simulink model "ADCS_r2017b"  (R2018a)
settings: Solver=FixedStepAuto  StartTime=0.0  StopTime=end_time  FixedStep=delta_t  RelTol=1e-3
undefined symbols (not defined in the file or in its folder): delta_t, SC, SS
libraries: sharedutil x5, vrlib x2
(part 2 of 3)

== system ADCS_r2017b/Satellite Simulator/Kinematics/Position Kinematics/Adams Bashforth Integration2 ==
  x_initial : Inport
  x_dot : Inport  Port=2
  dt : Inport  Port=3
  Delay : Delay  DelayLength=1  InitialConditionSource=Input port  InitialCondition=0
      settings: InputPortMap=u0,p4
  Delay1 : Delay  DelayLength=1  InitialConditionSource=Input port  InitialCondition=0
      settings: InputPortMap=u0,p4
  Delay2 : Delay  DelayLength=1  InitialConditionSource=Input port  InitialCondition=0
      settings: InputPortMap=u0,p4
  Gain : Gain  Gain=23/12
  Gain1 : Gain  Gain=-16/12
  Gain2 : Gain  Gain=5/12
  Product : Product
  Sum : Sum  Inputs=|++
  Sum1 : Sum  Inputs=+++
  x : Outport
  wires:
  x_initial/1 -> Delay/2
  Delay/1 -> Sum/1
  Sum/1 -> Delay/1, x/1
  Delay1/1 -> Delay2/1, Gain1/1
  x_dot/1 -> Delay2/2, Delay1/2, Delay1/1, Gain/1
  Gain1/1 -> Sum1/2
  Gain/1 -> Sum1/1
  Gain2/1 -> Sum1/3
  Sum1/1 -> Product/1
  dt/1 -> Product/2
  Product/1 -> Sum/2
  Delay2/1 -> Gain2/1

== system ADCS_r2017b/Satellite Simulator/Kinematics/Rotation Kinematics/Adams Bashforth Integration ==
  x_initial : Inport
  x_dot : Inport  Port=2
  dt : Inport  Port=3
  Delay : Delay  DelayLength=1  InitialConditionSource=Input port  InitialCondition=0
      settings: InputPortMap=u0,p4
  Delay1 : Delay  DelayLength=1  InitialConditionSource=Input port  InitialCondition=0
      settings: InputPortMap=u0,p4
  Delay2 : Delay  DelayLength=1  InitialConditionSource=Input port  InitialCondition=0
      settings: InputPortMap=u0,p4
  Gain : Gain  Gain=23/12
  Gain1 : Gain  Gain=-16/12
  Gain2 : Gain  Gain=5/12
  Product : Product
  Quaternion Normalize : sharedutil/Quaternion Normalize
      settings: SourceProductName=Aerospace Blockset  SourceProductBaseCode=AE
  Sum : Sum  Inputs=|++
  Sum1 : Sum  Inputs=+++
  x : Outport
  wires:
  x_initial/1 -> Delay/2
  Delay/1 -> Sum/1
  Sum/1 -> Quaternion Normalize/1
  Delay1/1 -> Delay2/1, Gain1/1
  x_dot/1 -> Delay2/2, Delay1/2, Delay1/1, Gain/1
  Gain1/1 -> Sum1/2
  Gain/1 -> Sum1/1
  Gain2/1 -> Sum1/3
  Sum1/1 -> Product/1
  dt/1 -> Product/2
  Product/1 -> Sum/2
  Delay2/1 -> Gain2/1
  Quaternion Normalize/1 -> Delay/1, x/1

== system ADCS_r2017b/Satellite Simulator/Kinematics/Rotation Kinematics/Adams Bashforth Integration1 ==
  x_initial : Inport
  x_dot : Inport  Port=2
  dt : Inport  Port=3
  Delay : Delay  DelayLength=1  InitialConditionSource=Input port  InitialCondition=0
      settings: InputPortMap=u0,p4
  Delay1 : Delay  DelayLength=1  InitialConditionSource=Input port  InitialCondition=0
      settings: InputPortMap=u0,p4
  Delay2 : Delay  DelayLength=1  InitialConditionSource=Input port  InitialCondition=0
      settings: InputPortMap=u0,p4
  Gain : Gain  Gain=23/12
  Gain1 : Gain  Gain=-16/12
  Gain2 : Gain  Gain=5/12
  Product : Product
  Sum : Sum  Inputs=|++
  Sum1 : Sum  Inputs=+++
  x : Outport
  wires:
  x_initial/1 -> Delay/2
  Delay/1 -> Sum/1
  Sum/1 -> Delay/1, x/1
  Delay1/1 -> Delay2/1, Gain1/1
  x_dot/1 -> Delay2/2, Delay1/2, Delay1/1, Gain/1
  Gain1/1 -> Sum1/2
  Gain/1 -> Sum1/1
  Gain2/1 -> Sum1/3
  Sum1/1 -> Product/1
  dt/1 -> Product/2
  Product/1 -> Sum/2
  Delay2/1 -> Gain2/1

== system ADCS_r2017b/Flight Software/Subsystems/RCS Controller/3 Axis Controller/Controller ==
  q_est : Inport
  w_est : Inport  Port=2
  q_target : Inport  Port=3
  w_target : Inport  Port=4
  gains : Inport  Port=5
  Constant : Constant  Value=[0;0;0;0;0;0;0;0;0;0;0;0]
  Terminator{,1..4} (5 alike) : Terminator
  RCS Cmd : Outport
  wires:
  q_est/1 -> Terminator/1
  w_est/1 -> Terminator1/1
  q_target/1 -> Terminator2/1
  w_target/1 -> Terminator3/1
  Constant/1 -> RCS Cmd/1
  gains/1 -> Terminator4/1

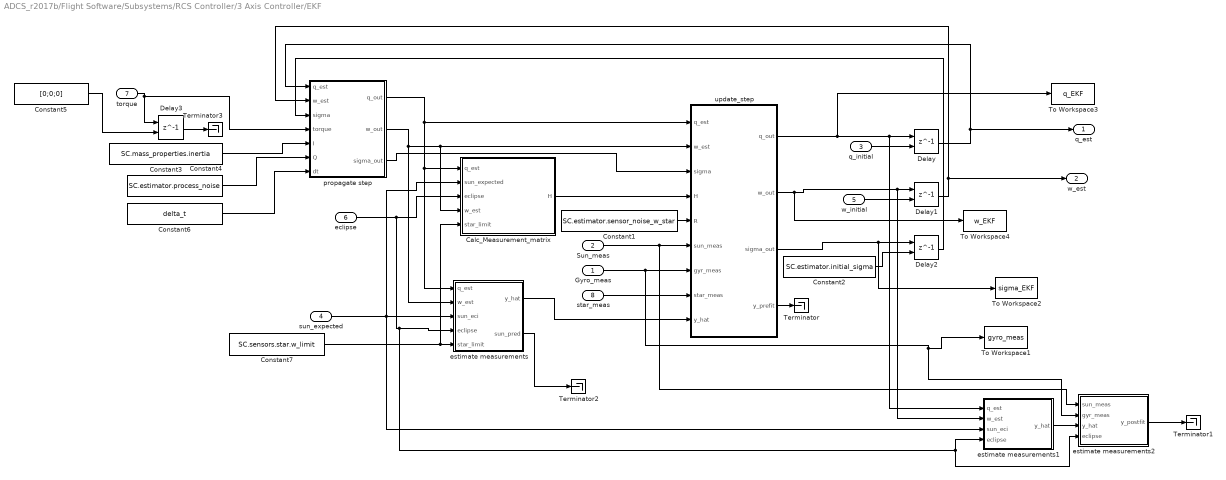
== system ADCS_r2017b/Flight Software/Subsystems/RCS Controller/3 Axis Controller/EKF ==
  Gyro_meas : Inport
  Sun_meas : Inport  Port=2
  q_initial : Inport  Port=3
  sun_expected : Inport  Port=4
  w_initial : Inport  Port=5
  eclipse : Inport  Port=6
  torque : Inport  Port=7
  star_meas : Inport  Port=8
  Calc_Measurement_matrix : MATLAB Function  TreatAsAtomicUnit=on
  Constant1 : Constant  Value=SC.estimator.sensor_noise_w_star
  Constant2 : Constant  Value=SC.estimator.initial_sigma
  Constant3 : Constant  Value=SC.mass_properties.inertia
  Constant4 : Constant  Value=SC.estimator.process_noise
  Constant5 : Constant  Value=[0;0;0]
  Constant6 : Constant  Value=delta_t
  Constant7 : Constant  Value=SC.sensors.star.w_limit
  Delay{,1..3} (4 alike) : Delay  DelayLength=1  InitialConditionSource=Input port  InitialCondition=0
      settings: InputPortMap=u0,p4
  Terminator{,1..3} (4 alike) : Terminator
  To Workspace1 : ToWorkspace  VariableName=gyro_meas  SampleTime=-1
  To Workspace2 : ToWorkspace  VariableName=sigma_EKF  SampleTime=-1
  To Workspace3 : ToWorkspace  VariableName=q_EKF  SampleTime=-1
  To Workspace4 : ToWorkspace  VariableName=w_EKF  SampleTime=-1
  estimate measurements : MATLAB Function  TreatAsAtomicUnit=on
  estimate measurements1 : MATLAB Function  TreatAsAtomicUnit=on
  estimate measurements2 : MATLAB Function  TreatAsAtomicUnit=on
  propagate step : MATLAB Function  TreatAsAtomicUnit=on
  update_step : MATLAB Function  TreatAsAtomicUnit=on
  q_est : Outport
  w_est : Outport  Port=2
  wires:
  Constant3/1 -> propagate step/5(I)
  sun_expected/1 -> estimate measurements/3(sun_eci), Calc_Measurement_matrix/2(sun_expected), estimate measurements1/3(sun_eci)
  Delay2/1 -> propagate step/3(sigma)
  Constant6/1 -> propagate step/7(dt)
  estimate measurements/1(y_hat) -> update_step/9(y_hat)
  q_initial/1 -> Delay/2
  estimate measurements2/1(y_postfit) -> Terminator1/1
  eclipse/1 -> estimate measurements/4(eclipse), estimate measurements1/4(eclipse), estimate measurements2/4(eclipse), Calc_Measurement_matrix/3(eclipse)
  update_step/2(w_out) -> To Workspace4/1, estimate measurements1/2(w_est), Delay1/1
  Delay1/1 -> w_est/1, propagate step/2(w_est)
  Constant4/1 -> propagate step/6(Q)
  update_step/1(q_out) -> To Workspace3/1, estimate measurements1/1(q_est), Delay/1
  w_initial/1 -> Delay1/2
  propagate step/2(w_out) -> Calc_Measurement_matrix/4(w_est), update_step/2(w_est), estimate measurements/2(w_est)
  propagate step/1(q_out) -> update_step/1(q_est), estimate measurements/1(q_est), Calc_Measurement_matrix/1(q_est)
  estimate measurements/2(sun_pred) -> Terminator2/1
  Delay/1 -> q_est/1, propagate step/1(q_est)
  Constant1/1 -> update_step/5(R)
  Calc_Measurement_matrix/1(H) -> update_step/4(H)
  Constant2/1 -> Delay2/2
  propagate step/3(sigma_out) -> update_step/3(sigma)
  Sun_meas/1 -> estimate measurements2/1(sun_meas), update_step/6(sun_meas)
  update_step/3(sigma_out) -> To Workspace2/1, Delay2/1
  Gyro_meas/1 -> To Workspace1/1, estimate measurements2/2(gyr_meas), update_step/7(gyr_meas)
  estimate measurements1/1(y_hat) -> estimate measurements2/3(y_hat)
  torque/1 -> propagate step/4(torque), Delay3/1
  Constant5/1 -> Delay3/2
  Constant7/1 -> Calc_Measurement_matrix/5(star_limit), estimate measurements/5(star_limit)
  star_meas/1 -> update_step/8(star_meas)
  update_step/4(y_prefit) -> Terminator/1
  Delay3/1 -> Terminator3/1

== system ADCS_r2017b/Flight Software/Subsystems/RCS Controller/3 Axis Controller/State Estimator ==
  gyro : Inport
  sun : Inport  Port=2
  star : Inport  Port=3
  Sun_eci_expected : Inport  Port=4
  Deterministic : Subsystem
  Q Method : Subsystem
  Subsystem : Subsystem
  To Workspace : ToWorkspace  VariableName=q_est_det  SampleTime=-1
  To Workspace1 : ToWorkspace  VariableName=w_est_det  SampleTime=-1
  To Workspace2 : ToWorkspace  VariableName=q_est_q  SampleTime=-1
  To Workspace3 : ToWorkspace  VariableName=w_est_q  SampleTime=-1
  To Workspace4 : ToWorkspace  VariableName=q_est_int  SampleTime=-1
  To Workspace5 : ToWorkspace  VariableName=w_est_int  SampleTime=-1
  q_est : Outport
  w_est : Outport  Port=2
  wires:
  gyro/1 -> Subsystem/1(w_body), Q Method/2(gyro), Deterministic/1(gyro)
  star/1 -> Q Method/3(star), Deterministic/2(star)
  sun/1 -> Q Method/1(sun_dir)
  Deterministic/1(q_est) -> To Workspace/1
  Deterministic/2(w_est) -> To Workspace1/1
  Q Method/1(q_est) -> To Workspace2/1, q_est/1
  Q Method/2(w_est) -> To Workspace3/1, w_est/1
  Subsystem/1(q_est) -> To Workspace4/1
  Subsystem/2(w_est) -> To Workspace5/1
  Sun_eci_expected/1 -> Q Method/4(sun_exp)

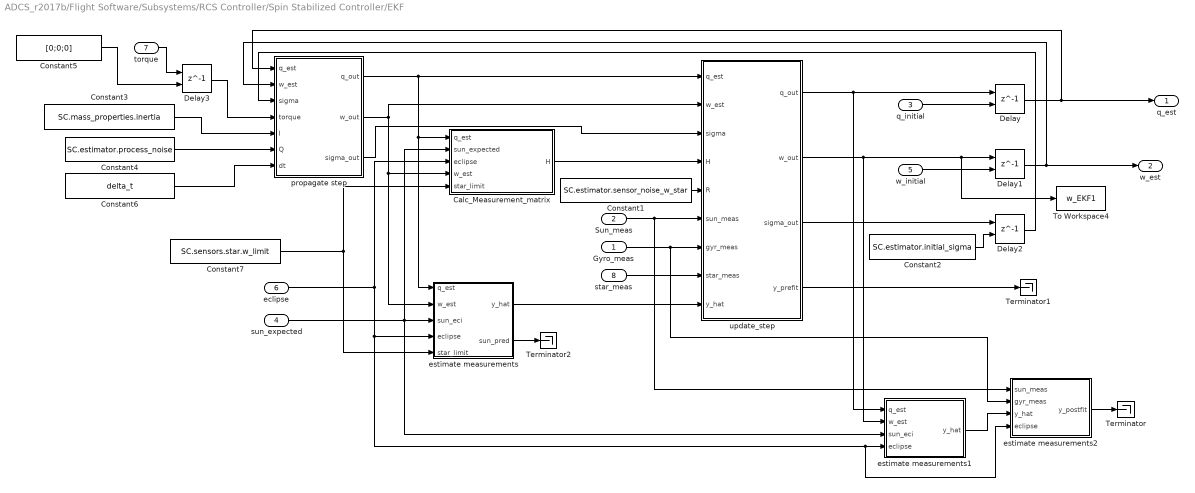
== system ADCS_r2017b/Flight Software/Subsystems/RCS Controller/Spin Stabilized Controller/EKF ==
  Gyro_meas : Inport
  Sun_meas : Inport  Port=2
  q_initial : Inport  Port=3
  sun_expected : Inport  Port=4
  w_initial : Inport  Port=5
  eclipse : Inport  Port=6
  torque : Inport  Port=7
  star_meas : Inport  Port=8
  Calc_Measurement_matrix : MATLAB Function  TreatAsAtomicUnit=on
  Constant1 : Constant  Value=SC.estimator.sensor_noise_w_star
  Constant2 : Constant  Value=SC.estimator.initial_sigma
  Constant3 : Constant  Value=SC.mass_properties.inertia
  Constant4 : Constant  Value=SC.estimator.process_noise
  Constant5 : Constant  Value=[0;0;0]
  Constant6 : Constant  Value=delta_t
  Constant7 : Constant  Value=SC.sensors.star.w_limit
  Delay{,1..3} (4 alike) : Delay  DelayLength=1  InitialConditionSource=Input port  InitialCondition=0
      settings: InputPortMap=u0,p4
  Terminator : Terminator
  Terminator1 : Terminator
  Terminator2 : Terminator
  To Workspace4 : ToWorkspace  VariableName=w_EKF1  SampleTime=-1
  estimate measurements : MATLAB Function  TreatAsAtomicUnit=on
  estimate measurements1 : MATLAB Function  TreatAsAtomicUnit=on
  estimate measurements2 : MATLAB Function  TreatAsAtomicUnit=on
  propagate step : MATLAB Function  TreatAsAtomicUnit=on
  update_step : MATLAB Function  TreatAsAtomicUnit=on
  q_est : Outport
  w_est : Outport  Port=2
  wires:
  Constant3/1 -> propagate step/5(I)
  sun_expected/1 -> Calc_Measurement_matrix/2(sun_expected), estimate measurements/3(sun_eci), estimate measurements1/3(sun_eci)
  Delay2/1 -> propagate step/3(sigma)
  Constant6/1 -> propagate step/7(dt)
  estimate measurements/1(y_hat) -> update_step/9(y_hat)
  q_initial/1 -> Delay/2
  estimate measurements2/1(y_postfit) -> Terminator/1
  eclipse/1 -> Calc_Measurement_matrix/3(eclipse), estimate measurements2/4(eclipse), estimate measurements1/4(eclipse), estimate measurements/4(eclipse)
  update_step/2(w_out) -> estimate measurements1/2(w_est), To Workspace4/1, Delay1/1
  Delay1/1 -> propagate step/2(w_est), w_est/1
  Constant4/1 -> propagate step/6(Q)
  update_step/4(y_prefit) -> Terminator1/1
  update_step/1(q_out) -> estimate measurements1/1(q_est), Delay/1
  w_initial/1 -> Delay1/2
  propagate step/2(w_out) -> update_step/2(w_est), Calc_Measurement_matrix/4(w_est), estimate measurements/2(w_est)
  propagate step/1(q_out) -> update_step/1(q_est), estimate measurements/1(q_est), Calc_Measurement_matrix/1(q_est)
  Delay/1 -> propagate step/1(q_est), q_est/1
  Constant1/1 -> update_step/5(R)
  Calc_Measurement_matrix/1(H) -> update_step/4(H)
  Constant2/1 -> Delay2/2
  propagate step/3(sigma_out) -> update_step/3(sigma)
  Sun_meas/1 -> update_step/6(sun_meas), estimate measurements2/1(sun_meas)
  update_step/3(sigma_out) -> Delay2/1
  Gyro_meas/1 -> update_step/7(gyr_meas), estimate measurements2/2(gyr_meas)
  estimate measurements1/1(y_hat) -> estimate measurements2/3(y_hat)
  Delay3/1 -> propagate step/4(torque)
  torque/1 -> Delay3/1
  Constant5/1 -> Delay3/2
  estimate measurements/2(sun_pred) -> Terminator2/1
  star_meas/1 -> update_step/8(star_meas)
  Constant7/1 -> estimate measurements/5(star_limit), Calc_Measurement_matrix/5(star_limit)

== system ADCS_r2017b/Flight Software/Subsystems/RCS Controller/3 Axis Controller/State Estimator/Deterministic ==
  gyro : Inport
  star : Inport  Port=2
  q_est : Outport
  w_est : Outport  Port=2
  wires:
  star/1 -> q_est/1
  gyro/1 -> w_est/1

== system ADCS_r2017b/Flight Software/Subsystems/RCS Controller/3 Axis Controller/State Estimator/Q Method ==
  sun_dir : Inport
  gyro : Inport  Port=2
  star : Inport  Port=3
  sun_exp : Inport  Port=4
  Constant : Constant  Value=SC.sensors.weights
  q_method : MATLAB Function  TreatAsAtomicUnit=on
  q_est : Outport  PortDimensions=4
  w_est : Outport  Port=2
  wires:
  sun_dir/1 -> q_method/2(sun_meas)
  q_method/1(q) -> q_est/1
  gyro/1 -> w_est/1
  star/1 -> q_method/3(q_body)
  sun_exp/1 -> q_method/1(sun_expected)
  Constant/1 -> q_method/4(weights)

== system ADCS_r2017b/Flight Software/Subsystems/RCS Controller/3 Axis Controller/State Estimator/Subsystem ==
  w_body : Inport
  Adams Bashforth Integration : Subsystem  TreatAsAtomicUnit=on
  Constant : Constant  Value=SC.initial_state.q
  Constant2 : Constant  Value=delta_t
  Delay : Delay  DelayLength=1  InitialConditionSource=Input port  InitialCondition=0
      settings: InputPortMap=u0,p4
  calc_q_dot : MATLAB Function  TreatAsAtomicUnit=on
  q_est : Outport
  w_est : Outport  Port=2
  wires:
  calc_q_dot/1(q_dot) -> Adams Bashforth Integration/2(x_dot)
  w_body/1 -> w_est/1, calc_q_dot/2(w)
  Constant/1 -> Delay/2, Adams Bashforth Integration/1(x_initial)
  Delay/1 -> calc_q_dot/1(q)
  Constant2/1 -> Adams Bashforth Integration/3(dt)
  Adams Bashforth Integration/1(x) -> Delay/1, q_est/1

== system ADCS_r2017b/Flight Software/Subsystems/RCS Controller/3 Axis Controller/State Estimator/Subsystem/Adams Bashforth Integration ==
  x_initial : Inport
  x_dot : Inport  Port=2
  dt : Inport  Port=3
  Delay : Delay  DelayLength=1  InitialConditionSource=Input port  InitialCondition=0
      settings: InputPortMap=u0,p4
  Delay1 : Delay  DelayLength=1  InitialConditionSource=Input port  InitialCondition=0
      settings: InputPortMap=u0,p4
  Delay2 : Delay  DelayLength=1  InitialConditionSource=Input port  InitialCondition=0
      settings: InputPortMap=u0,p4
  Gain : Gain  Gain=23/12
  Gain1 : Gain  Gain=-16/12
  Gain2 : Gain  Gain=5/12
  Product : Product
  Quaternion Normalize : sharedutil/Quaternion Normalize
      settings: SourceProductName=Aerospace Blockset  SourceProductBaseCode=AE
  Sum : Sum  Inputs=|++
  Sum1 : Sum  Inputs=+++
  x : Outport
  wires:
  x_initial/1 -> Delay/2
  Delay/1 -> Sum/1
  Sum/1 -> Quaternion Normalize/1
  Delay1/1 -> Delay2/1, Gain1/1
  x_dot/1 -> Delay2/2, Delay1/2, Delay1/1, Gain/1
  Gain1/1 -> Sum1/2
  Gain/1 -> Sum1/1
  Gain2/1 -> Sum1/3
  Sum1/1 -> Product/1
  dt/1 -> Product/2
  Product/1 -> Sum/2
  Delay2/1 -> Gain2/1
  Quaternion Normalize/1 -> Delay/1, x/1

== matlab function ADCS_r2017b/Flight Software/Subsystems/Sensor Processing/Process Gyro ==
  data: raw input; gyro output; gain input; offset input; rot input
function gyro = process_gyro(raw, gain, offset, rot)

temp = rot * raw;
gyro = gain .* (temp - offset);

== matlab function ADCS_r2017b/Flight Software/Subsystems/Mode Selection/MATLAB Function ==
  data: Kp output; gyro input; Kd output; eclipse input; JD input; mode output; ax3_gains input; ax3_TC input; spin_gains input; spin_TC input; spin_up_gains input; spin_up_TC input
function [Kp, Kd, mode]  = Mode_Logic(gyro, eclipse, JD, ax3_gains, ax3_TC, spin_gains, spin_TC, spin_up_gains, spin_up_TC)
%JD_i = 2458610.000; %initial JD
JD_i = 2458611.2081011; %actual initial JD
minutes_elapsed = (JD-JD_i)*(24*60);

if(minutes_elapsed < 10)
    mode = 0; %de-tumble controller
elseif(minutes_elapsed < 20)
    mode = 1; %three axis control
elseif(minutes_elapsed < 30)
    mode = 3; %spin controller
else
    mode = 4; %uncontrolled
end

if mode == 0
    Kp = 0*ax3_gains(1:3);
    Kd = ax3_gains(4:6);
elseif mode == 1
    Kp = ax3_gains(1:3);
    Kd = ax3_gains(4:6);
elseif mode == 2
    Kp = spin_up_gains(1:3);
    Kd = spin_up_gains(4:6);
elseif mode == 3
    Kp = spin_gains(1:3);
    Kd = spin_gains(4:6);
else
    Kp = [0;0;0];
    Kd = [0;0;0];
end
    
end

== matlab function ADCS_r2017b/Flight Software/Subsystems/Sensor Processing/Process Gyro1 ==
  data: raw input; sun_dir output; gain input; offset input; eclipse output; threshold input
function [sun_dir, eclipse] = process_sun(raw, gain, offset, threshold)
n = length(raw); %number of sun sensors
sun = zeros(n,1);
for i=1:length(raw)
    sun(i) = gain(i) * (raw(i) - offset(i));
end

%discuss advantages of different ways of turning sun measurements to direction
sun_x = sun(1)-sun(2);
sun_y = sun(3)-sun(4);
sun_z = sun(5)-sun(6);

sun_dir = [sun_x; sun_y; sun_z];
sun_dir = sun_dir/norm(sun_dir);

eclipse = 0;
if (sum(abs(sun)) < threshold)
    eclipse = 1;
    sun_dir = [0;0;0];
end

== matlab function ADCS_r2017b/Satellite Simulator/Kinematics/Backup Rotation Kinematics/Euler Equations ==
  data: w input; w_dot output; tor input; I input
function w_dot = fcn(w, tor, I)

w_dot = -I\(Skew(w)*I*w-tor);

% w_dot = zeros(size(w));
% wx = w(1); wy = w(2); wz = w(3);
% Ix = I(1,1); Iy = I(2,2); Iz = I(3,3);
% w_dot(1) = (tor(1) - (Iz-Iy)*wx*wz)/Ix;  %update this to work in body axis
% w_dot(2) = (tor(2) - (Ix-Iz)*wz*wx)/Iy;
% w_dot(3) = (tor(3) - (Iy-Ix)*wx*wy)/Iz;
end


function S = Skew(v)
S = [0 -v(3) v(2)
    v(3) 0 -v(1)
    -v(2) v(1) 0];
end

== matlab function ADCS_r2017b/Satellite Simulator/Kinematics/Backup Rotation Kinematics/calc_e_dot ==
  data: e input; e_dot output; w input
function e_dot   = calc_e_dot( e, w )
%INPUT: euler angles, angular velocity
%OUTPUT: rate of change of euler angles
%propagate actual dynamics
    tan_the = tan(e(2));
    if(abs(tan_the) > 300) %make sure tan(theta) is well defined
        tan_the = 300*sign(tan_the);
        disp('tan x')
    end
    cos_the = cos(e(2));
    if(abs(cos_the) < 10^-4) %make sure cos(theta) is well defined
        cos_the = 10^-4*sign(cos_the);
        disp('cos x')
    end
    A = [1, tan_the*sin(e(1)), tan_the*cos(e(1));
         0, cos(e(1)),              -1*sin(e(1));
         0, sin(e(1))/cos_the,  cos(e(1))/cos_the];
    e_dot = A*w;
end

== matlab function ADCS_r2017b/Satellite Simulator/External Forces and Torques/External Forces/MATLAB Function ==
  data: srp input; srp_tot output
function srp_tot = fcn(srp)
%srp_tot = zeros(3,1);
%srp is 3x6
srp_tot = sum(srp, 2);
%srp_tot = [0;0;0];

== matlab function ADCS_r2017b/Satellite Simulator/Kinematics/Calc Coordinate Transforms/Calc_R_eci2body ==
  data: q input; R_eci2body output
function R_eci2body = fcn(q)
eta=q(4);
e1=q(1);
e2=q(2);
e3=q(3);

R_eci2body = [e1^2-e2^2-e3^2+eta^2, 2*(e1*e2+eta*e3),        2*(e1*e3-eta*e2);
              2*(e1*e2-eta*e3),     -1*e1^2+e2^2-e3^2+eta^2, 2*(e2*e3+eta*e1);
              2*(e1*e3+eta*e2),     2*(e2*e3-eta*e1),        -1*e1^2-e2^2+e3^2+eta^2];
          
end

== matlab function ADCS_r2017b/Satellite Simulator/External Forces and Torques/External Torques/MATLAB Function ==
  data: r_mci input; y output; r_moon input
function y = fcn(r_mci, r_moon)

y = (norm(r_mci) < 0.9*r_moon);

== matlab function ADCS_r2017b/Satellite Simulator/Kinematics/Calc Coordinate Transforms/Calc_R_eci2ecef ==
  data: JD_i input; R_eci2ecef output
function R_eci2ecef = fcn(JD_i)
%Based on Seidlemann's "Explanatory Supplment to the Astronomical Almanac" page 50
%Given the JD, will return the rotation matrix to convert R_eci to R_ecef
JD = floor(JD_i);
seconds_per_day = 24*60*60;
SSN = seconds_per_day*(JD_i-JD);
seconds_per_half_day = seconds_per_day/2;
days_per_Julian_century = 36525;
JD_epoch = 2451545.00; %JD of noon on Jan 1, 2000

c1 = JD-JD_epoch+(SSN/seconds_per_day);
c2 = c1/days_per_Julian_century;

p1 = 24110.54841;
p2 = 8640184.812866;
p3 = 0.093104;
p4 = -6.2*10^-6;

c3 = (p1)+(p2*c2)+(p3*c2*c2)+(p4*c2*c2*c2)+(SSN)-(seconds_per_half_day);

c4 = c3*pi/seconds_per_half_day;

c5 = mod(c4, 2*pi);

a1 = cos(c5);
a2 = sin(c5);
a3 = -1*a2;
a4 = 0;
a5 = 1;
A = [a1;a3;a4;a2;a1;a4;a4;a4;a5];

R_eci2ecef = reshape(A, 3,3);
end

== matlab function ADCS_r2017b/Satellite Simulator/Kinematics/Calc Coordinate Transforms/ecef2geod ==
  data: h output; r_ecef input; phi output; lambda output
function [h,phi,lambda] = ecef2geod(r_ecef)
%note - r_ecef should be in meters
a = 6378137;        %earth radius, meters
e = 0.081819190842; %earth eccentricity

% Reference: function ecef2geodetic in Matlab
x = r_ecef(1);
y = r_ecef(2);
z = r_ecef(3);

% Ellipsoid constants
e2 = e ^ 2;   % Square of first eccentricity
ep2 = e2 / (1 - e2);     % Square of second eccentricity
f = 1 - sqrt(1 - e2);    % Flattening
b = a * (1 - f);         % Semiminor axis
% Longitude
lambda = atan2(y,x); %[rad]
% Distance from Z-axis
rho = hypot(x,y);
% Bowring's formula for initial parametric (beta) and geodetic (phi) latitudes
beta = atan2(z, (1 - f) * rho);
phi = atan2(z   + b * ep2 * sin(beta).^3,...
            rho - a * e2  * cos(beta).^3); %[rad]
% Fixed-point iteration with Bowring's formula
% (typically converges within two or three iterations)
betaNew = atan2((1 - f)*sin(phi), cos(phi));
count = 0;
while any(beta ~= betaNew) && count < 5
    beta = betaNew;
    phi = atan2(z   + b * ep2 * sin(beta).^3,...
                rho - a * e2  * cos(beta).^3);
    betaNew = atan2((1 - f)*sin(phi), cos(phi));
    count = count + 1;
end
% Calculate ellipsoidal height from the final value for latitude
sinphi = sin(phi);
N = a ./ sqrt(1 - e2 * sinphi.^2);
h = rho .* cos(phi) + (z + e2 * N .* sinphi) .* sinphi - N;

phi=phi*180/pi; %[deg]
lambda=lambda*180/pi; %[deg]
end

== matlab function ADCS_r2017b/Satellite Simulator/Kinematics/Rotation Kinematics/calc_q_dot ==
  data: q input; q_dot output; w input
function q_dot   = fcn(q, w)

wx = w(1); wy = w(2); wz = w(3);
OMEGA = [   0,    wz, -1*wy, wx;
        -1*wz,     0,    wx, wy;
           wy, -1*wx,     0, wz;
        -1*wx, -1*wy, -1*wz,  0];
q_dot = 0.5*OMEGA*q;

== matlab function ADCS_r2017b/Satellite Simulator/Environment/Subsystem/MATLAB Function ==
  data: decYear input; B_ned output; yearLastEpoch input; lastgh input; ghslope input; latitude input; longitude input; altitude input
function B_ned  = igrf_mag_field(decYear, yearLastEpoch, lastgh, ghslope, latitude, longitude, altitude)
% IGRF Earth's magnetic field from IGRF model.
% 
% Usage: B = IGRF(COEFS, LATITUDE, LONGITUDE, ALTITUDE)
% 
% Calculates the components of the Earth's magnetic field using the
% International Geomagnetic Reference Field (IGRF) model. The inputs for
% the position can be scalars.
% 
% When all the coordinate inputs are scalars, the function can be run more
% efficiently by providing the proper IGRF coefficient vector for a given
% time rather than the time itself. This mode is useful when making
% multiple calls to the function while keeping the time the same (meaning
% the coefficients will be the same for each run) as loading the
% coefficients can be the most time-consuming part of the function. The
% coefficient vector can be easily loaded using the function LOADIGRFCOEFS.
% This mode is assumed when all the coordinate inputs are scalars and the
% first input is a vector. In this case, the coefficient vector should be
% formatted as (LOADIGRFCOEFS provides this):
% 
%   [g(n=1,m=0) g(n=1,m=1) h(n=1,m=1) g(n=2,m=0) g(n=2,m=1) h(n=2,m=1) ...]
% 
% Regardless of the size of the inputs, the outputs will be column vectors.
% If only one output is requested, B = [BX(:), BY(:), BZ(:)] is output.
% Note that the other parameters the IGRF gives can be computed from BX,
% BY, and BZ as:
% 
%   Horizonal intensity: hypot(BX, BY) (i.e., sqrt(BX.^2 + BY.^2) )
%   Total intensity: hypot(BX, hypot(BY, BZ))
%   Declination: atan2(BY, BX)
%   Inclination: atan(BZ./hypot(BX, BY))
% 
% This function relies on having the file igrfcoefs.mat in the MATLAB
% path to function properly when a time is input. If this file cannot be
% found, this function will try to create it by calling GETIGRFCOEFS.
% 
% The IGRF is a spherical harmonic expansion of the Earth's internal
% magnetic field. Currently, the IGRF model is valid between the years 1900
% and 2015. See the health warning for the IGRF model here:
% http://www.ngdc.noaa.gov/IAGA/vmod/igrfhw.html
% 
% Reference:
% International Association of Geomagnetism and Aeronomy, Working Group 
% V-MOD (2010), International Geomagnetic Reference Field: the eleventh
% generation, _Geophys. J. Int._, _183_(3), 1216-1230, 
% doi:10.1111/j.1365-246X.2010.04804.x.
% 
% Inputs:
%   -COEFS: Instead of inputting a time, you can simply specify the proper
%   coefficients for the time you want by inputting in the first argument
%   the proper coefficient vector from igrfcoefs.mat.
%   -LATITUDE: Geocentric or geodetic latitude in degrees.
%   -LONGITUDE: Geocentric or geodetic longitude in degrees.
%   -ALTITUDE: For geodetic coordiates, the height in km above the Earth's
%   surface. For geocentric coordiates, the radius in km from the center of
%   the Earth.

% 
% Outputs:
%   -BX: Northward component of the magnetic field in nanoteslas (nT).
%   -BY: Eastward component of the magnetic field in nT.
%   -BZ: Downward component of the magnetic field in nT.
%   -B: [BX(:), BY(:), BZ(:)].
% 
% See also: LOADIGRFCOEFS, GETIGRFCOEFS, IGRFLINE, DATENUM, IGRF11MAGM.


%%%%%%%%%%%%%%%%%%%%%%%%%%%%%%%%%%%%%%%%%%%%%%%%%%%%%%%%%%%%%%%%%%%%%%%%%%%
%%%%%%%%%%%%%%%%%%%        IGRF scalar function.        %%%%%%%%%%%%%%%%%%%
%%%%%%%%%%%%%%%%%%%%%%%%%%%%%%%%%%%%%%%%%%%%%%%%%%%%%%%%%%%%%%%%%%%%%%%%%%%
%function [Bx, By, Bz] = igrfs(time, latitude, longitude, altitude, coord)

% Fundamental constant.
Rearth_km = 6371.2;
altitude=altitude/1000;
%%% SPHERICAL COORDINATE CONVERSION %%%
% Convert the latitude, longitude, and altitude coordinates input into
% spherical coordinates r (radius), theta (inclination angle from +z axis),
% and phi (azimuth angle from +x axis).
% We want cos(theta) and sin(theta) rather than theta itself.
costheta = cos((90 - latitude)*pi/180);
sintheta = sin((90 - latitude)*pi/180);

% Convert from geodetic coordinates to geocentric coordinates if necessary.
% This method was adapted from igrf11syn, which was a conversion of the
% IGRF subroutine written in FORTRAN.

    a = 6378.137; f = 1/298.257223563; b = a*(1 - f);
    rho = hypot(a*sintheta, b*costheta);
    r = sqrt( altitude.^2 + 2*altitude.*rho + ...
        (a^4*sintheta.^2 + b^4*costheta.^2) ./ rho.^2 );
    cd = (altitude + rho) ./ r;
    sd = (a^2 - b^2) ./ rho .* costheta.*sintheta./r;
    oldcos = costheta;
    costheta = costheta.*cd - sintheta.*sd;
    sintheta = sintheta.*cd + oldcos.*sd;


% Convert longitude to radians.
phi = longitude*pi/180;

%%% GET PROPER IGRF COEFFICIENTS %%%

gh=lastgh+ghslope*(decYear-yearLastEpoch);
nmax = sqrt(numel(gh) + 1) - 1;


% We need cos(m*phi) and sin(m*phi) multiple times, so precalculate into a
% vector here:
cosphi = cos((1:nmax)*phi);
sinphi = sin((1:nmax)*phi);

Pmax = (nmax+1)*(nmax+2)/2;

%%% BEGIN MAGNETIC FIELD CALCULATION %%%
% Initialize variables used in for loop below.
Br = 0; Bt = 0; Bp = 0;
 P = zeros(1, Pmax);  P(1) = 1;  P(3) = sintheta;
dP = zeros(1, Pmax); dP(1) = 0; dP(3) = costheta;

% For this initial condition, the first if will result in n = 1, m = 0.
m = 1; n = 0; coefindex = 1;

a_r = (Rearth_km/r)^2;

% Increment through all the n's and m's. gh will be a vector with g
% followed by h for incrementing through n and m except when h would be
% redundant (i.e., when m = 0).
for Pindex = 2:Pmax
    
    % Increment to the next n when m becomes larger than n.
    if n < m
        m = 0;
        n = n + 1;
        a_r = a_r*(Rearth_km/r); % We need (Rearth_km./r)^(n+2)
    end
    
    % Calculate P and dP. They are given recursively according to:
    % 
    % P(0, 0) = 1, P(1, 1) = sin(theta) <- Specified above
    % P(n, n) = sqrt(1 - 1/(2n))*sin(theta)*P(n-1, n-1)
    % P(n, m) = (2n - 1)/sqrt(n^2 - m^2)*cos(theta)*P(n-1, m) -
    %     sqrt(((n-1)^2 - m^2) / (n^2 - m^2)) * P(n-2, m)
    % 
    % dP(0, 0) = 0, dP(1, 1) = cos(theta) <- Specified above
    % dP(n, n) = sqrt(1 - 1/(2n))*(sin(theta)*dP(n-1, n-1) +
    %     cos(theta)*P(n-1, n-1))
    % dP(n, m) = (2n - 1)/sqrt(n^2 - m^2)*(cos(theta)*dP(n-1, m) -
    %     sin(theta)*P(n-1, m)) - sqrt(((n-1)^2 - m^2)/(n^2 - m^2))*
    %     dP(n-2, m)
    if m < n && Pindex ~= 3 % (Pindex=3 is n=1, m=1, initial cond. above)
        last1n = Pindex - n;
        last2n = Pindex - 2*n + 1;
        P(Pindex) = (2*n - 1)/sqrt(n^2 - m^2)*costheta*P(last1n) - ...
            sqrt(((n-1)^2 - m^2) / (n^2 - m^2)) * P(last2n);
        dP(Pindex) = (2*n - 1)/sqrt(n^2 - m^2)*(costheta*dP(last1n) - ...
            sintheta*P(last1n)) - sqrt(((n-1)^2 - m^2) / (n^2 - m^2)) * ...
            dP(last2n);
    elseif Pindex ~= 3
        lastn = Pindex - n - 1;
        P(Pindex) = sqrt(1 - 1/(2*m))*sintheta*P(lastn);
        dP(Pindex) = sqrt(1 - 1/(2*m))*(sintheta*dP(lastn) + ...
            costheta*P(lastn));
    end
    
    % Calculate the magnetic field components as a running sum. Find
    % explicit expressions for these in Global Earth Physics: a Handbook of
    % Physical Constants by Thomas J. Aherns (1995), pg. 49. Link:
    % http://books.google.com/books?id=aqjU_NHyre4C&lpg=PP1&dq=Global%20
    % earth%20physics%3A%20a%20handbook%20of%20physical%20constants&pg=PA49
    % #v=onepage&q&f=false
    % (except equation 6 is missing a required 1/sin(theta) and m; correct
    % equations on page 5 (equations 3a-3c) of:
    % http://hanspeterschaub.info/Papers/UnderGradStudents/
    % MagneticField.pdf)
    if m == 0 % Implies h = 0, so only coefficient in gh is g
        coef = a_r*gh(coefindex); %*cos(0*phi) = 1
        Br = Br + (n+1)*coef*P(Pindex);
        Bt = Bt - coef*dP(Pindex);
        % Bp is 0 for m = 0.
        coefindex = coefindex + 1; % Only need to skip over g this time.
    else
        coef = a_r*(gh(coefindex)*cosphi(m) + gh(coefindex+1)*sinphi(m));
        Br = Br + (n+1)*coef*P(Pindex);
        Bt = Bt - coef*dP(Pindex);
        if sintheta == 0 % Use different formula when dividing by 0.
            Bp = Bp - costheta*a_r*(-gh(coefindex)*sinphi(m) + ...
                gh(coefindex+1)*cosphi(m))*dP(Pindex);
        else
            Bp = Bp - 1/sintheta*a_r*m*(-gh(coefindex)*sinphi(m) + ...
                gh(coefindex+1)*cosphi(m))*P(Pindex);
        end
        coefindex = coefindex + 2; % Skip over g and h this time.
    end
    
    % Increment m.
    m = m + 1;
    
end

% Convert from spherical to (x,y,z) = (North,East,Down).
Bx = -Bt;
By = Bp;
Bz = -Br;

% Convert back to geodetic coordinates if necessary.
Bx_old = Bx;
Bx = Bx.*cd + Bz.*sd;
Bz = Bz.*cd - Bx_old.*sd;

B_ned = [Bx;By;Bz];

== matlab function ADCS_r2017b/Satellite Simulator/Kinematics/Calc Coordinate Transforms/MATLAB Function ==
  data: lati input; R_ecef2ned output; long input
function R_ecef2ned   = calc_ECEF_to_NED( lati, long )
%Given the latitude and longitude, returns the rotation matrix to tranform
%ECEF coordinates into NED coordinates.
%   Detailed explanation goes here
phi = lati*pi/180; %radians
lam = long*pi/180; %radians
sinp = sin(phi);
sinl = sin(lam);
cosp = cos(phi);
cosl = cos(lam);

A = zeros(3,3);
A(1,1) = -1*sinp*cosl;
A(1,2) = -1*sinp*sinl;
A(1,3) =    cosp;
A(2,1) = -1*sinl;
A(2,2) =    cosl;
A(2,3) = 0;
A(3,1) = -1*cosp*cosl;
A(3,2) = -1*cosp*sinl;
A(3,3) = -1*sinp;

R_ecef2ned = A;
end

== matlab function ADCS_r2017b/Satellite Simulator/Kinematics/Calc Coordinate Transforms/Calc_R_eci2mci ==
  data: obliq_e input; R_eci2mci output; obliq_m input
function R_eci2mci = fcn(obliq_e, obliq_m)
ang = (pi/180) * (obliq_e - obliq_m);

%check if this needs to be -1*ang
R_eci2mci = [1,0,0;
             0,cos(ang),-1*sin(ang);
             0,sin(ang),   cos(ang)];
end

== matlab function ADCS_r2017b/Satellite Simulator/External Forces and Torques/External Torques/Grav gradient earth/MATLAB Function ==
  data: rIr input; tor output; r_eci input; GM input
function tor = fcn(rIr, r_eci, GM)
r = norm(r_eci);
tor = (3*GM)/(r^3) * rIr;
end

== matlab function ADCS_r2017b/Satellite Simulator/External Forces and Torques/External Torques/Grav gradient moon/MATLAB Function ==
  data: rIr input; tor output; r_mci input; GM input
function tor = fcn(rIr, r_mci, GM)
r = norm(r_mci);
tor = (3*GM)/(r^3) * rIr;

== matlab function ADCS_r2017b/Flight Software/Subsystems/RCS Controller/3 Axis Controller/Calc_R_eci2mci ==
  data: obliq_e input; R_eci2mci output; obliq_m input
function R_eci2mci = fcn(obliq_e, obliq_m)
ang = (pi/180) * (obliq_e - obliq_m);

%check if this needs to be -1*ang
R_eci2mci = [1,0,0;
             0,cos(ang),-1*sin(ang);
             0,sin(ang),   cos(ang)];
end

== matlab function ADCS_r2017b/Satellite Simulator/Actuators/RCS Model ==
  data: command input; force_body output; torque_body output; moment_arm input; norm_dir input; max_thrust input; noise input; bias input
function [force_body, torque_body] = fcn(command, moment_arm, norm_dir, max_thrust, noise, bias)
%input: 12 commands, on range from 0-1, corresponding to which thruster to fir
 force_body = [0;0;0];
torque_body = [0;0;0];
num = length(command); %number of thrusters, should be 12.

for i=1:num
    ax = bias(i,1); ay = bias(i,2); az = bias(i,3);
    R_bias = [    1,    az, -1*ay;
              -1*az,     1,    ax;
                 ay, -1*ax,     1];
    dt = 1 + noise*randn(1,1);
     force_body =  force_body - dt*max_thrust*command(i)*R_bias*norm_dir(:,i);
    torque_body = torque_body + dt*max_thrust*command(i)*cross(R_bias*norm_dir(:,i),moment_arm(:,i));
end

== matlab function ADCS_r2017b/Flight Software/Subsystems/RCS Controller/3 Axis Controller/dcm2quat ==
  data: R_mci2eci input; q output
function q = dcm2quat(R_mci2eci)
% eta=q(4);
% e1=q(1);
% e2=q(2);
% e3=q(3);
% 
% R_eci2body = [e1^2-e2^2-e3^2+eta^2, 2*(e1*e2+eta*e3),        2*(e1*e3-eta*e2);
%               2*(e1*e2-eta*e3),     -1*e1^2+e2^2-e3^2+eta^2, 2*(e2*e3+eta*e1);
%               2*(e1*e3+eta*e2),     2*(e2*e3-eta*e1),        -1*e1^2-e2^2+e3^2+eta^2];
   
A = R_mci2eci;
%q_temp = zeros(4,1);
%q_temp = dcm2quat(R_mci2eci);
%q = [q_temp(2:4), q_temp(1)]';
q4 = 0.5*sqrt(1+A(1,1) + A(2,2) + A(3,3));
q1 = (A(2,3) - A(3,2))/(4*q4);
q2 = (A(3,1) - A(1,3))/(4*q4);
q3 = (A(1,2) - A(2,1))/(4*q4);
q = [q1;q2;q3;q4];
end

== matlab function ADCS_r2017b/Flight Software/Subsystems/RCS Controller/Environment/Sun position in ECI ==
  data: JD_tt input; sun_eci output; moon_eci input; sol_emb_eph_coeff input; sol_sun_eph_coeff input; sol_sun_jd_lookup input
function sun_eci   = calc_sun_pos(JD_tt, moon_eci, sol_emb_eph_coeff, sol_sun_eph_coeff, sol_sun_jd_lookup)
%calculate the position of the sun in the eci frame based on the lookup
%coefficients and table provided.
persistent coeff2;
persistent fract_v2;

if(JD_tt > sol_sun_jd_lookup(end))
    disp('Error, JD is past final sun table value.')
end

%index and fraction of JD
k = -1;
f = -1;
for(i=1:length(sol_sun_jd_lookup-1))
    if(JD_tt >= sol_sun_jd_lookup(i) && JD_tt <= sol_sun_jd_lookup(i+1))
        k = i;
        f = (JD_tt-sol_sun_jd_lookup(i))/(sol_sun_jd_lookup(i+1)-sol_sun_jd_lookup(i)); %f in range 0,1
        break
    end
end
f = 2*f-1; %fraction scaled in valid range -1,1
if(k<0)    %past end of table, k never reset
    k = length(sol_sun_jd_lookup)-1;
    f = 1;
end
%cheby
order = 12;
y = zeros(order+1,1);
if(isempty(coeff2))
    coeff2 = zeros(order+1, order+1);
    coeff2(1,1) = 1;
    coeff2(2,2) = 1;
    for(idx = 3:order+1)
        coeff2(idx,:) = 2*[0 coeff2(idx-1,1:end-1)]-coeff2(idx-2,:);
    end
    fract_v2 = zeros(order+1,1);
    fract_v2(1) = 1;
end

y(1) = 1;
for(ind = 2:order+1)
    fract_v2(ind) = fract_v2(ind-1)*f;
    for(sub_ind = ind:-2:1)
        y(ind) = y(ind)+fract_v2(sub_ind)*coeff2(ind,sub_ind);
    end
end
y11 = y(1:11);

coeff_x1 = sol_emb_eph_coeff(k,  1:13);
coeff_y1 = sol_emb_eph_coeff(k, 14:26);
coeff_z1 = sol_emb_eph_coeff(k, 27:39);

coeff_x2 = sol_sun_eph_coeff(k,  1:11);
coeff_y2 = sol_sun_eph_coeff(k, 12:22);
coeff_z2 = sol_sun_eph_coeff(k, 23:33);

moon_pos = 0.012150585609624*moon_eci;

sun_eci = [0;0;0];
sun_eci(1) = 1000*dot(coeff_x1, y);
sun_eci(2) = 1000*dot(coeff_y1, y);
sun_eci(3) = 1000*dot(coeff_z1, y);

sun_eci = sun_eci-moon_pos;

sun_eci(1) = 1000*dot(coeff_x2, y11)-sun_eci(1);
sun_eci(2) = 1000*dot(coeff_y2, y11)-sun_eci(2);
sun_eci(3) = 1000*dot(coeff_z2, y11)-sun_eci(3);

end

== matlab function ADCS_r2017b/Flight Software/Subsystems/RCS Controller/Environment/Moon position in ECI ==
  data: JD_tt input; moon_eci output; mop_moon_eph_coeff input; mop_moon_jd_lookup input
function moon_eci   = calc_moon_pos(JD_tt, mop_moon_eph_coeff, mop_moon_jd_lookup)
%calculate the position of the moon in the eci frame based on the lookup
%coefficients and table provided.
persistent coeff;
persistent fract_v;

if(JD_tt > mop_moon_jd_lookup(end))
    disp('Error, JD is past final moon table value.')
end

%index and fraction of JD
k = -1;
f = -1;
for(i=1:length(mop_moon_jd_lookup-1))
    if(JD_tt >= mop_moon_jd_lookup(i) && JD_tt <= mop_moon_jd_lookup(i+1))
        k = i;
        f = (JD_tt-mop_moon_jd_lookup(i))/(mop_moon_jd_lookup(i+1)-mop_moon_jd_lookup(i)); %f in range 0,1
        break
    end
end
f = 2*f-1; %fraction scaled in valid range -1,1
if(k<0)    %past end of table, k never reset
    k = length(mop_moon_jd_lookup)-1;
    f = 1;
end
%cheby
order = 12;
y = zeros(order+1,1);
if(isempty(coeff))
    coeff = zeros(order+1, order+1);
    coeff(1,1) = 1;
    coeff(2,2) = 1;
    for(idx = 3:order+1)
        coeff(idx,:) = 2*[0 coeff(idx-1,1:end-1)]-coeff(idx-2,:);
    end
    fract_v = zeros(order+1,1);
    fract_v(1) = 1;
end

y(1) = 1;
for(ind = 2:order+1)
    fract_v(ind) = fract_v(ind-1)*f;
    for(sub_ind = ind:-2:1)
        y(ind) = y(ind)+fract_v(sub_ind)*coeff(ind,sub_ind);
    end
end

coeff_x = mop_moon_eph_coeff(k,  1:13);
coeff_y = mop_moon_eph_coeff(k, 14:26);
coeff_z = mop_moon_eph_coeff(k, 27:39);

moon_eci =[0;0;0];
moon_eci(1) = 1000*dot(coeff_x, y);
moon_eci(2) = 1000*dot(coeff_y, y);
moon_eci(3) = 1000*dot(coeff_z, y);
end

== matlab function ADCS_r2017b/Flight Software/Subsystems/RCS Controller/3 Axis Controller/State Estimator/Q Method/q_method ==
  data: sun_expected input; q output; sun_meas input; q_body input; weights input
function q = fcn(sun_expected, sun_meas, q_body, weights)
%q_temp = [q_body(4), q_body(1:3)'];
%xyz_meas = quat2dcm(q_temp);
q_body = q_body / norm(q_body);
eta=q_body(4);
e1=q_body(1);
e2=q_body(2);
e3=q_body(3);

xyz_meas = [e1^2-e2^2-e3^2+eta^2, 2*(e1*e2+eta*e3),          2*(e1*e3-eta*e2);
              2*(e1*e2-eta*e3),     -1*e1^2+e2^2-e3^2+eta^2, 2*(e2*e3+eta*e1);
              2*(e1*e3+eta*e2),     2*(e2*e3-eta*e1),        -1*e1^2-e2^2+e3^2+eta^2];
x_m = xyz_meas(:,1);
y_m = xyz_meas(:,2);
z_m = xyz_meas(:,3);
x_b = [1;0;0];
y_b = [0;1;0];
z_b = [0;0;1];

s_m = sun_meas / norm(sun_meas);
s_b = sun_expected  / norm(sun_expected);
w = zeros(3,4);
w(:,1) = sqrt(weights(1)) * x_m;
w(:,2) = sqrt(weights(2)) * y_m;
w(:,3) = sqrt(weights(3)) * z_m;
w(:,4) = sqrt(weights(4)) * s_m;
u = zeros(3,4);
u(:,1) = sqrt(weights(1)) * x_b;
u(:,2) = sqrt(weights(2)) * y_b;
u(:,3) = sqrt(weights(3)) * z_b;
u(:,4) = sqrt(weights(4)) * s_b;

B = w * u';
S = B+B';
Z = [B(2,3)-B(3,2); B(3,1)-B(1,3); B(1,2)-B(2,1)];
sig = trace(B);
K = [ S-eye(3)*sig, Z;
       Z', sig];

[vec, val] = eig(K);
[~, ind] = max(max(val));
q = vec(:,ind);

== matlab function ADCS_r2017b/Flight Software/Subsystems/RCS Controller/3 Axis Controller/State Estimator/Subsystem/calc_q_dot ==
  data: q input; q_dot output; w input
function q_dot   = fcn(q, w)

wx = w(1); wy = w(2); wz = w(3);
OMEGA = [   0,    wz, -1*wy, wx;
        -1*wz,     0,    wx, wy;
           wy, -1*wx,     0, wz;
        -1*wx, -1*wy, -1*wz,  0];
q_dot = 0.5*OMEGA*q;

== matlab function ADCS_r2017b/Flight Software/Subsystems/RCS Controller/Spin Stabilized Controller/Controller ==
  data: R_mci2eci input; q_est input; tor output; w_est input; Kp input; Kd input; w_des input; mode input
function tor  = fcn(R_mci2eci, q_est, w_est, Kp, Kd, w_des, mode)
if(mode < 1.5)
    w_des = 0*w_des;
end

if(mode > 3.5)
    Kp = 0*Kp;
    Kd = 0*Kd;
end

As = quat2dcm(q_est); %aka R_eci2body
At = R_mci2eci';  %target

z_body = [0;0;1];
z_mci  = [0;0;1];
z_mci  = R_mci2eci * z_mci;
z_mci  = As * z_mci; %get z_mci in the body frame
alpha  = acos(z_mci(3) / norm(z_mci)); %dot(z_body, z_mci)
vec    = cross(z_body, z_mci/norm(z_mci));
q_tar = [vec(1)*sin(alpha/2); vec(2)*sin(alpha/2); vec(3)*sin(alpha/2); cos(alpha/2)];
At = quat2dcm(q_tar); %try this instead, AZ, 6/4/2019

%Ae = As * At';
Ae = At;

%Ae_dot = (Ae-Ae_prev)/0.1;

tor = zeros(3, 1);
% linear control for small errors
% alpha_x = Ae(2,3);
% alpha_y = Ae(3,1);
% alpha_z = Ae(1,2);
% tor(1) = -Kp*alpha_x -Kd*w_est(1);
% tor(2) = -Kp*alpha_y -Kd*w_est(2);
% tor(3) = -Kp*alpha_z -Kd*w_est(3);
%Kp = [0;0;0];
% non-linear control for larger errors

tor(1) = -Kp(1)*.5*(Ae(2,3) - Ae(3,2)) - Kd(1)*(w_est(1)-w_des(1));
tor(2) = -Kp(2)*.5*(Ae(3,1) - Ae(1,3)) - Kd(2)*(w_est(2)-w_des(2));
tor(3) = -Kp(3)*.5*(Ae(1,2) - Ae(2,1)) - Kd(3)*(w_est(3)-w_des(3));

% tor(1) = -Kp(1)*.5*(Ae(2,3) - Ae(3,2)) - Kd(1)*.5*(Ae_dot(2,3) - Ae_dot(3,2));
% tor(2) = -Kp(2)*.5*(Ae(3,1) - Ae(1,3)) - Kd(2)*.5*(Ae_dot(3,1) - Ae_dot(1,3));
% tor(3) = -Kp(3)*.5*(Ae(1,2) - Ae(2,1)) - Kd(3)*.5*(Ae_dot(1,2) - Ae_dot(2,1));
end

function R_eci2body = quat2dcm(q)
eta=q(4);
e1=q(1);
e2=q(2);
e3=q(3);

R_eci2body = [e1^2-e2^2-e3^2+eta^2, 2*(e1*e2+eta*e3),        2*(e1*e3-eta*e2);
              2*(e1*e2-eta*e3),     -1*e1^2+e2^2-e3^2+eta^2, 2*(e2*e3+eta*e1);
              2*(e1*e3+eta*e2),     2*(e2*e3-eta*e1),        -1*e1^2-e2^2+e3^2+eta^2];
          
end

function S = skew(v)
S = [0 -v(3) v(2)
    v(3) 0 -v(1)
    -v(2) v(1) 0];
end

== matlab function ADCS_r2017b/Satellite Simulator/Environment/Sun position in ECI ==
  data: JD_tt input; sun_eci output; moon_eci input; sol_emb_eph_coeff input; sol_sun_eph_coeff input; sol_sun_jd_lookup input
function sun_eci   = calc_sun_pos(JD_tt, moon_eci, sol_emb_eph_coeff, sol_sun_eph_coeff, sol_sun_jd_lookup)
%calculate the position of the sun in the eci frame based on the lookup
%coefficients and table provided.
persistent coeff2;
persistent fract_v2;

if(JD_tt > sol_sun_jd_lookup(end))
    disp('Error, JD is past final sun table value.')
end

%index and fraction of JD
k = -1;
f = -1;
for(i=1:length(sol_sun_jd_lookup-1))
    if(JD_tt >= sol_sun_jd_lookup(i) && JD_tt <= sol_sun_jd_lookup(i+1))
        k = i;
        f = (JD_tt-sol_sun_jd_lookup(i))/(sol_sun_jd_lookup(i+1)-sol_sun_jd_lookup(i)); %f in range 0,1
        break
    end
end
f = 2*f-1; %fraction scaled in valid range -1,1
if(k<0)    %past end of table, k never reset
    k = length(sol_sun_jd_lookup)-1;
    f = 1;
end
%cheby
order = 12;
y = zeros(order+1,1);
if(isempty(coeff2))
    coeff2 = zeros(order+1, order+1);
    coeff2(1,1) = 1;
    coeff2(2,2) = 1;
    for(idx = 3:order+1)
        coeff2(idx,:) = 2*[0 coeff2(idx-1,1:end-1)]-coeff2(idx-2,:);
    end
    fract_v2 = zeros(order+1,1);
    fract_v2(1) = 1;
end

y(1) = 1;
for(ind = 2:order+1)
    fract_v2(ind) = fract_v2(ind-1)*f;
    for(sub_ind = ind:-2:1)
        y(ind) = y(ind)+fract_v2(sub_ind)*coeff2(ind,sub_ind);
    end
end
y11 = y(1:11);

coeff_x1 = sol_emb_eph_coeff(k,  1:13);
coeff_y1 = sol_emb_eph_coeff(k, 14:26);
coeff_z1 = sol_emb_eph_coeff(k, 27:39);

coeff_x2 = sol_sun_eph_coeff(k,  1:11);
coeff_y2 = sol_sun_eph_coeff(k, 12:22);
coeff_z2 = sol_sun_eph_coeff(k, 23:33);

moon_pos = 0.012150585609624*moon_eci;

sun_eci = [0;0;0];
sun_eci(1) = 1000*dot(coeff_x1, y);
sun_eci(2) = 1000*dot(coeff_y1, y);
sun_eci(3) = 1000*dot(coeff_z1, y);

sun_eci = sun_eci-moon_pos;

sun_eci(1) = 1000*dot(coeff_x2, y11)-sun_eci(1);
sun_eci(2) = 1000*dot(coeff_y2, y11)-sun_eci(2);
sun_eci(3) = 1000*dot(coeff_z2, y11)-sun_eci(3);

end

== matlab function ADCS_r2017b/Satellite Simulator/Environment/Moon position in ECI ==
  data: JD_tt input; moon_eci output; mop_moon_eph_coeff input; mop_moon_jd_lookup input
function moon_eci   = calc_moon_pos(JD_tt, mop_moon_eph_coeff, mop_moon_jd_lookup)
%calculate the position of the moon in the eci frame based on the lookup
%coefficients and table provided.
persistent coeff;
persistent fract_v;

if(JD_tt > mop_moon_jd_lookup(end))
    disp('Error, JD is past final moon table value.')
end

%index and fraction of JD
k = -1;
f = -1;
for(i=1:length(mop_moon_jd_lookup-1))
    if(JD_tt >= mop_moon_jd_lookup(i) && JD_tt <= mop_moon_jd_lookup(i+1))
        k = i;
        f = (JD_tt-mop_moon_jd_lookup(i))/(mop_moon_jd_lookup(i+1)-mop_moon_jd_lookup(i)); %f in range 0,1
        break
    end
end
f = 2*f-1; %fraction scaled in valid range -1,1
if(k<0)    %past end of table, k never reset
    k = length(mop_moon_jd_lookup)-1;
    f = 1;
end
%cheby
order = 12;
y = zeros(order+1,1);
if(isempty(coeff))
    coeff = zeros(order+1, order+1);
    coeff(1,1) = 1;
    coeff(2,2) = 1;
    for(idx = 3:order+1)
        coeff(idx,:) = 2*[0 coeff(idx-1,1:end-1)]-coeff(idx-2,:);
    end
    fract_v = zeros(order+1,1);
    fract_v(1) = 1;
end

y(1) = 1;
for(ind = 2:order+1)
    fract_v(ind) = fract_v(ind-1)*f;
    for(sub_ind = ind:-2:1)
        y(ind) = y(ind)+fract_v(sub_ind)*coeff(ind,sub_ind);
    end
end

coeff_x = mop_moon_eph_coeff(k,  1:13);
coeff_y = mop_moon_eph_coeff(k, 14:26);
coeff_z = mop_moon_eph_coeff(k, 27:39);

moon_eci =[0;0;0];
moon_eci(1) = 1000*dot(coeff_x, y);
moon_eci(2) = 1000*dot(coeff_y, y);
moon_eci(3) = 1000*dot(coeff_z, y);
end

== matlab function ADCS_r2017b/Satellite Simulator/Environment/calc_eclipse ==
  data: sun_eci input; eclipse output; moon_eci input; r_eci input; R_eci2mci input
function eclipse = fcn(sun_eci, moon_eci, r_eci, R_eci2mci)

eclipse_earth = 0;
eclipse_moon  = 0;
sun_mci = R_eci2mci*(sun_eci - moon_eci);
  r_mci = R_eci2mci*( r_eci - moon_eci);

%check for ecclipse with earth
%ref: Vallado, page 201
R_e = 6378137;
f = 1/298.257223563;
e = sqrt(2*f-f*f);
d_sun = norm(sun_eci);
d_sat = norm(r_eci);
temp = 1/sqrt(1-e^2);
sun_eci(3) = sun_eci(3)*temp;
  r_eci(3) =   r_eci(3)*temp;
if (abs(d_sun^2 + d_sat^2 - 2*dot(sun_eci,r_eci)) < 0.0001)
    t_min = 0;
else
    t_min = (d_sun^2 - dot(sun_eci,r_eci)) / (d_sun^2+d_sat^2-2*dot(sun_eci,r_eci));
end

if ( t_min < 0 || t_min > 1)
    eclipse_earth = 0;
else
    distsqrd = ((1-t_min)*d_sun^2+t_min*dot(sun_eci,r_eci))/(R_e^2);
    if distsqrd > 1
        eclipse_earth = 0;
    else
        eclipse_earth = 1;
    end
end

%check for eclipse with moon
R_m = 1738100;
f = 0.0012;
e = sqrt(2*f-f*f);
d_sun = norm(sun_mci);
d_sat = norm(r_mci);
temp = 1/sqrt(1-e^2);
sun_mci(3) = sun_mci(3)*temp;
  r_mci(3) =   r_mci(3)*temp;
if (abs(d_sun^2 + d_sat^2 - 2*dot(sun_mci,r_mci)) < 0.0001)
    t_min = 0;
else
    t_min = (d_sun^2 - dot(sun_mci,r_mci)) / (d_sun^2+d_sat^2-2*dot(sun_mci,r_mci));
end

if ( t_min < 0 || t_min > 1)
    eclipse_moon = 0;
else
    distsqrd = ((1-t_min)*d_sun^2+t_min*dot(sun_mci,r_mci))/(R_m^2);
    if distsqrd > 1
        eclipse_moon = 0;
    else
        eclipse_moon = 1;
    end
end

%eclipse_earth = 0;
%eclipse_moon = 0;

if(eclipse_earth || eclipse_moon)
    eclipse = 1;
else
    eclipse = 0;
end

end

== matlab function ADCS_r2017b/Flight Software/Subsystems/RCS Controller/3 Axis Controller/Controller1 ==
  data: R_mci2eci input; q_est input; tor output; w_est input; Kp input; Kd input
function tor  = fcn(R_mci2eci, q_est, w_est, Kp, Kd)
As = quat2dcm(q_est);
At = R_mci2eci';

Ae = As * At';
%Ae_dot = (Ae-Ae_prev)/0.1;

tor = zeros(3, 1);
% linear control for small errors
% alpha_x = Ae(2,3);
% alpha_y = Ae(3,1);
% alpha_z = Ae(1,2);
% tor(1) = -Kp*alpha_x -Kd*w_est(1);
% tor(2) = -Kp*alpha_y -Kd*w_est(2);
% tor(3) = -Kp*alpha_z -Kd*w_est(3);
%Kp = [0;0;0];
% non-linear control for larger errors

tor(1) = -Kp(1)*.5*(Ae(2,3) - Ae(3,2)) - Kd(1)*(w_est(1));
tor(2) = -Kp(2)*.5*(Ae(3,1) - Ae(1,3)) - Kd(2)*(w_est(2));
tor(3) = -Kp(3)*.5*(Ae(1,2) - Ae(2,1)) - Kd(3)*(w_est(3));

% tor(1) = -Kp(1)*.5*(Ae(2,3) - Ae(3,2)) - Kd(1)*.5*(Ae_dot(2,3) - Ae_dot(3,2));
% tor(2) = -Kp(2)*.5*(Ae(3,1) - Ae(1,3)) - Kd(2)*.5*(Ae_dot(3,1) - Ae_dot(1,3));
% tor(3) = -Kp(3)*.5*(Ae(1,2) - Ae(2,1)) - Kd(3)*.5*(Ae_dot(1,2) - Ae_dot(2,1));
end

function R_eci2body = quat2dcm(q)
eta=q(4);
e1=q(1);
e2=q(2);
e3=q(3);

R_eci2body = [e1^2-e2^2-e3^2+eta^2, 2*(e1*e2+eta*e3),        2*(e1*e3-eta*e2);
              2*(e1*e2-eta*e3),     -1*e1^2+e2^2-e3^2+eta^2, 2*(e2*e3+eta*e1);
              2*(e1*e3+eta*e2),     2*(e2*e3-eta*e1),        -1*e1^2-e2^2+e3^2+eta^2];
          
end

function S = skew(v)
S = [0 -v(3) v(2)
    v(3) 0 -v(1)
    -v(2) v(1) 0];
end

== matlab function ADCS_r2017b/Satellite Simulator/External Forces and Torques/External Forces/Aero Drag ==
  data: r_eci input; a_body output; v_eci input; R_eci2body input; CD input
function a_body = fcn(r_eci, v_eci, R_eci2body, CD)

a_body = [0;0;0];
end

== matlab function ADCS_r2017b/Satellite Simulator/External Forces and Torques/External Forces/Earth Gravity ==
  data: r_eci input; a_Earth_eci output; GM_Earth input
function a_Earth_eci = accelPointMass(r_eci, GM_Earth)
a_Earth_eci = -GM_Earth*r_eci./norm(r_eci)^3;
%a_eci = [0;0;0];
end
